simulink model "Grid-Connected Photovoltaic Power System"  (R2024a)
settings: Solver=VariableStepAuto  StartTime=0.0  StopTime=5  RelTol=1e-3
undefined symbols (not defined in the file): D1, Delta
libraries: spsIGBTLib x7, spsThreePhaseVIMeasurementLib x4, spsSeriesRLCBranchLib x3, simulink x3, spsThreePhaseSeriesRLCBranchLib x2, spsThreePhaseTransformerTwoWindingsLib x2, spsVoltageMeasurementLib x2, spsDiodeLib x1, spsGroundLib x1, spsPVArrayLib x1, spsPWMGeneratorDCDCLib x1, spsSawtoothGeneratorLib x1
settings Model: Creator=suresh43  LastModifiedBy=aniru
settings RTWCC: GPUComputeCapability=3.5

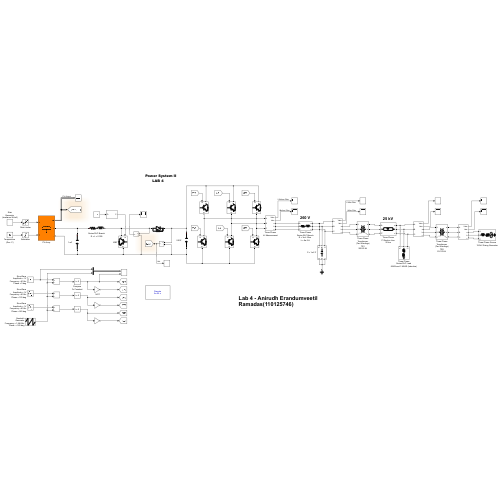
[thumbnail: Simulink's stored preview of the top-level diagram]
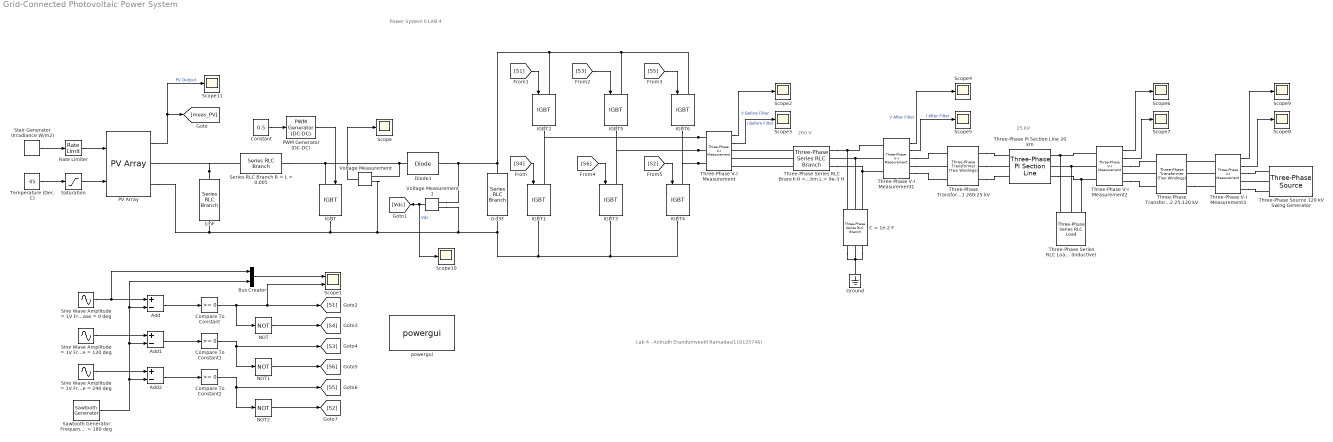
== system Grid-Connected Photovoltaic Power System ==
  note: Power System II
      | LAB 4
  note: 260 V
  note: 25 kV
  note: Lab 4 - Anirudh Erandumveetil Ramadas(110125746)
  0.05F : spsSeriesRLCBranchLib/Series RLC Branch  LConnTagsString=__new0  RConnTagsString=__new0  BranchType=C  Resistance=0  Inductance=0  SetiL0=off  InitialCurrent=0  Capacitance=0.05  Setx0=off  InitialVoltage=0  Measurements=None
  1mF : spsSeriesRLCBranchLib/Series RLC Branch  LConnTagsString=__new0  RConnTagsString=__new0  BranchType=C  Resistance=0  Inductance=0  SetiL0=off  InitialCurrent=0  Capacitance=1e-3  Setx0=off  InitialVoltage=0  Measurements=None
  Add : Sum  Inputs=+-
  Add1 : Sum  Inputs=+-
  Add2 : Sum  Inputs=+-
  Bus Creator : BusCreator  Inputs=2
  C = 1e-2 F : spsThreePhaseSeriesRLCBranchLib/Three-Phase Series RLC Branch  LConnTagsString=A|B|C  RConnTagsString=A|B|C  BranchType=C  Resistance=3e-4  Inductance=9e-5  Capacitance=1e-2  Measurements=None
  Compare To Constant : simulink/Logic and Bit Operations/Compare To Constant  relop=>=  const=0  OutDataTypeStr=boolean
  Compare To Constant1 : simulink/Logic and Bit Operations/Compare To Constant  relop=>=  const=0  OutDataTypeStr=boolean
  Compare To Constant2 : simulink/Logic and Bit Operations/Compare To Constant  relop=>=  const=0  OutDataTypeStr=boolean
  Constant : Constant  Value=0.5
  Diode1 : spsDiodeLib/Diode  Ron=1e-4  Lon=0  Vf=0  IC=0  UseSnubber=0  Rs=500  Cs=250e-9  Measurements=off
  Ground : spsGroundLib/Ground  LConnTagsString=a
  IGBT{,1..6} (7 alike) : spsIGBTLib/IGBT  Ron=0.001  Lon=0  Vf=1  Tf=1e-6  Tt=2e-6  IC=0  Rs=1e5  Cs=inf  Measurements=off
  NOT : Logic  Operator=NOT  IconShape=distinctive  AllPortsSameDT=off  OutDataTypeStr=boolean
  NOT1 : Logic  Operator=NOT  IconShape=distinctive  AllPortsSameDT=off  OutDataTypeStr=boolean
  NOT2 : Logic  Operator=NOT  IconShape=distinctive  AllPortsSameDT=off  OutDataTypeStr=boolean
  PV Array : spsPVArrayLib/PV Array  Npar=48  Nser=7  PlotType=array @ 25 deg.C & specified irradiances  S_vec=[ 1000 ]  Temp_C_vec="[ 45 25  ]"  ModuleName=SunPower SPR-305E-WHT-D  PlotWhenSelected=off  Pm=305.226  Ncell=96  Voc=64.2  Isc=5.96  Vm=54.7  Im=5.58  beta_Voc_pc=-0.2727  alpha_Isc_pc=0.061745  beta_Voc=-0.17507  alpha_Isc=0.00368  IL=5.9657  I0=6.3076e-12  nI=0.94489  Rsh=393.2054  Rs=0.37428  RobustModel=off  RobustCellTemperature=313.3991  BAL=on  Tc=1e-6  Tfilter=5e-5
  PWM Generator (DC-DC) : spsPWMGeneratorDCDCLib/PWM Generator (DC-DC)  Fsw=5e3  Ts=0
  Rate Limiter : RateLimiter  RisingSlewLimit=8000  FallingSlewLimit=-8000  SampleTimeMode=inherited  InitialCondition=1000
  Saturation : Saturate  UpperLimit=55  LowerLimit=5
  Sawtooth Generator Frequency = 1.98 KHz Phase  = 180 deg : spsSawtoothGeneratorLib/Sawtooth Generator  Freq=5000  Phase=180  Ts=0
  Scope{,2..11} (11 alike) : Scope
  Scope1 : Scope  NumInputPorts=2
  Series RLC Branch R = L = 0.005 : spsSeriesRLCBranchLib/Series RLC Branch  LConnTagsString=__new0  RConnTagsString=__new0  BranchType=RL  Resistance=0.005  Inductance=0.005  SetiL0=off  InitialCurrent=0  Capacitance=1e-6  Setx0=off  InitialVoltage=0  Measurements=None
  Sine Wave Amplitude = 1V Frequency = 60 Hz Phase = 0 deg : Sin  Frequency=376.991118  SampleTime=0
  Sine Wave Amplitude = 1V Frequency = 60 Hz Phase = 120 deg : Sin  Frequency=376.991118  Phase=-2.0944  SampleTime=0
  Sine Wave Amplitude = 1V Frequency = 60 Hz Phase = 240 deg : Sin  Frequency=376.991118  Phase=2.0944  SampleTime=0
  Stair Generator (Irradiance W/m2) : spsStairGeneratorLib/Stair Generator  t=[0, 0.4]  e=[0.5, 1]*1000  Ts=5e-5
  Temperature (Dec. C) : Constant  Value=45
  Three-Phase PI Section Line 20 km : spsThreePhasePISectionLineLib/Three-Phase PI Section Line  LConnTagsString=a|b|c  RConnTagsString=A|B|C  Length=20  Frequency=60  Resistances=[ 0.01273 0.3864]  Inductances="[ 0.9337e-3  4.1264e-3]"  Capacitances=[12.74e-9 7.751e-9]
  Three-Phase Series RLC Branch R = 3e-4 Ohm L = 9e-3 H : spsThreePhaseSeriesRLCBranchLib/Three-Phase Series RLC Branch  LConnTagsString=A|B|C  RConnTagsString=A|B|C  BranchType=RL  Resistance=3e-4  Inductance=9e-5  Capacitance=1e-6  Measurements=None
  Three-Phase Series RLC Load 8 MW and 1 MVAR (Inductive) : spsThreePhaseSeriesRLCLoadLib/Three-Phase Series RLC Load  LConnTagsString=A|B|C  Configuration=Y (grounded)  NominalVoltage=25e3  Vabc=[1e3 1e3 1e3]  Vabcp=[1e3 1e3 1e3]  NominalFrequency=60  UnbalancedPower=off  ActivePower=8e6  InductivePower=1e6  CapacitivePower=0  Pabc=[10e3 9e3 11e3]  QLabc=[100 90 110]  QCabc=[100 90 110]  Pabcp=[10e3 9e3 11e3]  QLabcp=[100 90 110]  QCabcp=[100 90 110]  Measurements=None  LoadType=constant Z
  Three-Phase Transformer (Two Windings) TR1 260:25 kV : spsThreePhaseTransformerTwoWindingsLib/Three-Phase Transformer (Two Windings)  Winding1Connection=Delta (D1)  Winding2Connection=Yg  CoreType=Three single-phase transformers  SetSaturation=off  Hysteresis=off  DataFile='hysteresis'  SetInitialFlux=off  Measurements=None  UNITS=pu  NominalPower=[ 100e3 , 60 ]  Winding1=[ 260 , 0.0012 , 0.03 ]  Winding2=[ 25e3 ,0.0012 , 0.03 ]  Rm=500  Lm=500  L0=0.5  Saturation=[ 0,0 ; 0.0024,1.2 ; 1.0,1.52 ]  InitialFluxes=[ 0.8 , -0.8 , 0.7 ]  BreakLoop=off  DiscreteSolver=Trapezoidal iterative  DataType=off  TransfoNumber=1
  Three-Phase Transformer (Two Windings) TR2 25:120 kV : spsThreePhaseTransformerTwoWindingsLib/Three-Phase Transformer (Two Windings)  Winding1Connection=Delta (D1)  Winding2Connection=Yg  CoreType=Three single-phase transformers  SetSaturation=off  Hysteresis=off  DataFile='hysteresis'  SetInitialFlux=off  Measurements=None  UNITS=pu  NominalPower=[ 10e6 , 60 ]  Winding1=[ 25e3 , 0.003 , 0.08 ]  Winding2=[ 120e3 ,0.003 , 0.08 ]  Rm=500  Lm=500  L0=0.5  Saturation=[ 0,0 ; 0.0024,1.2 ; 1.0,1.52 ]  InitialFluxes=[ 0.8 , -0.8 , 0.7 ]  BreakLoop=off  DiscreteSolver=Trapezoidal iterative  DataType=off  TransfoNumber=1
  Three-Phase V-I Measurement{,1..3} (4 alike) : spsThreePhaseVIMeasurementLib/Three-Phase V-I Measurement  VoltageMeasurement=phase-to-ground  SetLabelV=off  LabelV=Vabc  Vpu=off  VpuLL=off  CurrentMeasurement=yes  SetLabelI=off  LabelI=Iabc  Ipu=off  Pbase=100e6  Vbase=500e3  OutputType=Complex  PhasorSimulation=off  PSBequivalent=0
  "Three-Phase Source 120 kV Swing Generator " : spsThreePhaseSourceLib/Three-Phase Source  InternalConnection=Yg  VoltagePhases=off  Voltage=120e3  PhaseAngle=0  Voltage_phases=[25e3 25e3 25e3]/sqrt(3)  PhaseAngles_phases=[0 -120 +120]  Frequency=60  NonIdealSource=on  SpecifyImpedance=on  Resistance=0.8929  Inductance=16.58e-3  ShortCircuitLevel=100e6  BaseVoltage=120e3  XRratio=30  BusType=swing  Pref=10e3  Qref=0  Prefabc=[10e3, 10e3, 10e3]  Qrefabc=[0, 0, 0]  Qmin=-inf  Qmax=inf
  Voltage Measurement : spsVoltageMeasurementLib/Voltage Measurement  PhasorSimulation=off  OutputType=Complex  PSBequivalent=0
  Voltage Measurement1 : spsVoltageMeasurementLib/Voltage Measurement  PhasorSimulation=off  OutputType=Complex  PSBequivalent=0
  powergui : sps_lib/powergui  Priority=1  SimulationMode=Discrete  SampleTime=5e-5  frequency=60  Iterations=50  frequencyindice=0  Pbase=100e6  ErrMax=1e-4  UnitsV=kV  UnitsW=MW  buscounter=0  FunctionMessages=off  echomessages=off  EnableUseOfTLC=off  CurrentSourceSwitches=off  DisableSnubberDevices=off  DisableRonSwitches=off  DisableVfSwitches=off  DisplayEquations=off  AutomaticDiscreteSolvers=off  SolverType=Tustin/Backward Euler (TBE)  Interpol=off  ExternalGateDelay=off  methode=off  Ts=100  x0status=blocks  SPID=on  SwTol=0  HookPort=off  NonlinearTolerance=1e-4  nMaxIteration=100  ContinueOnMaxIteration=off  RestoreLinks=warning  ResistiveCurrentMeasurement=off  Frange=[0:2:500]  Ylog=off  Xlog=on  ShowGrid=off  save=off  variable=ZData  structure=0  ZoomFFT=off  StartTime=0.0  cycles=1  DisplayStyle=1  fundamental=60  FreqAxis=off  MaxFrequency=1000  frequencyindicesteady=1  RmsSteady=1  display=off
  wires:
  Temperature (Dec. C)/1 -> Saturation/1
  Saturation/1 -> PV Array/2
  Stair Generator (Irradiance W/m2)/1 -> Rate Limiter/1
  Rate Limiter/1 -> PV Array/1
  PV Array/1 -> Scope11/1, [meas_PV]  "PV Output"
  Constant/1 -> PWM Generator (DC-DC)/1
  PWM Generator (DC-DC)/1 -> IGBT/1
  Voltage Measurement/1 -> Scope/1
  Voltage Measurement1/1 -> Scope10/1, [Vdc]  "Vdc"
  [S4] -> IGBT1/1
  [S1] -> IGBT2/1
  [S3] -> IGBT5/1
  [S5] -> IGBT6/1
  [S6] -> IGBT3/1
  [S2] -> IGBT4/1
  Sawtooth Generator Frequency = 1.98 KHz Phase  = 180 deg/1 -> Add2/2, Add1/2, Bus Creator/2, Add/2
  Sine Wave Amplitude = 1V Frequency = 60 Hz Phase = 0 deg/1 -> Bus Creator/1, Add/1
  Sine Wave Amplitude = 1V Frequency = 60 Hz Phase = 120 deg/1 -> Add1/1
  Sine Wave Amplitude = 1V Frequency = 60 Hz Phase = 240 deg/1 -> Add2/1
  Add/1 -> Compare To Constant/1
  Add1/1 -> Compare To Constant1/1
  Add2/1 -> Compare To Constant2/1
  Compare To Constant/1 -> Scope1/2, [S1], NOT/1
  Compare To Constant1/1 -> [S3], NOT1/1
  Compare To Constant2/1 -> [S5], NOT2/1
  Bus Creator/1 -> Scope1/1
  NOT/1 -> [S4]
  NOT1/1 -> [S6]
  NOT2/1 -> [S2]
  Three-Phase V-I Measurement/1 -> Scope2/1  "V Before Filter"
  Three-Phase V-I Measurement/2 -> Scope3/1  "I Before Filter"
  Three-Phase V-I Measurement1/1 -> Scope4/1  "V After Filter"
  Three-Phase V-I Measurement1/2 -> Scope5/1  "I After Filter"
  Three-Phase V-I Measurement2/1 -> Scope6/1
  Three-Phase V-I Measurement2/2 -> Scope7/1
  Three-Phase V-I Measurement3/2 -> Scope8/1
  Three-Phase V-I Measurement3/1 -> Scope9/1
  connections:
  1mF/LConn1 -- Series RLC Branch R = L = 0.005/LConn1 -- PV Array/RConn1
  PV Array/RConn2 -- IGBT/RConn1 -- Voltage Measurement1/LConn2 -- IGBT1/RConn1 -- IGBT4/RConn1 -- IGBT3/RConn1 -- 0.05F/RConn1 -- Voltage Measurement/LConn2 -- 1mF/RConn1
  Series RLC Branch R = L = 0.005/RConn1 -- IGBT/LConn1 -- Voltage Measurement/LConn1 -- Diode1/LConn1
  Diode1/RConn1 -- Voltage Measurement1/LConn1 -- IGBT2/LConn1 -- IGBT6/LConn1 -- IGBT5/LConn1 -- 0.05F/LConn1
  Three-Phase V-I Measurement/LConn2 -- IGBT5/RConn1 -- IGBT3/LConn1
  Three-Phase V-I Measurement/LConn1 -- IGBT2/RConn1 -- IGBT1/LConn1
  Three-Phase V-I Measurement/LConn3 -- IGBT6/RConn1 -- IGBT4/LConn1
  Three-Phase Series RLC Branch R = 3e-4 Ohm L = 9e-3 H/LConn3 -- Three-Phase V-I Measurement/RConn3
  Three-Phase Series RLC Branch R = 3e-4 Ohm L = 9e-3 H/LConn2 -- Three-Phase V-I Measurement/RConn2
  Three-Phase Series RLC Branch R = 3e-4 Ohm L = 9e-3 H/LConn1 -- Three-Phase V-I Measurement/RConn1
  Three-Phase V-I Measurement1/LConn2 -- C = 1e-2 F/LConn2 -- Three-Phase Series RLC Branch R = 3e-4 Ohm L = 9e-3 H/RConn2
  Three-Phase Series RLC Branch R = 3e-4 Ohm L = 9e-3 H/RConn1 -- Three-Phase V-I Measurement1/LConn1 -- C = 1e-2 F/LConn1
  Three-Phase Series RLC Branch R = 3e-4 Ohm L = 9e-3 H/RConn3 -- Three-Phase V-I Measurement1/LConn3 -- C = 1e-2 F/LConn3
  Ground/LConn1 -- C = 1e-2 F/RConn3 -- C = 1e-2 F/RConn1 -- C = 1e-2 F/RConn2
  Three-Phase V-I Measurement1/RConn1 -- Three-Phase Transformer (Two Windings) TR1 260:25 kV/LConn1
  Three-Phase V-I Measurement1/RConn2 -- Three-Phase Transformer (Two Windings) TR1 260:25 kV/LConn2
  Three-Phase V-I Measurement1/RConn3 -- Three-Phase Transformer (Two Windings) TR1 260:25 kV/LConn3
  Three-Phase Transformer (Two Windings) TR1 260:25 kV/RConn2 -- Three-Phase PI Section Line 20 km/LConn2
  Three-Phase Transformer (Two Windings) TR1 260:25 kV/RConn1 -- Three-Phase PI Section Line 20 km/LConn1
  Three-Phase Transformer (Two Windings) TR1 260:25 kV/RConn3 -- Three-Phase PI Section Line 20 km/LConn3
  Three-Phase V-I Measurement2/LConn2 -- Three-Phase Series RLC Load 8 MW and 1 MVAR (Inductive)/LConn2 -- Three-Phase PI Section Line 20 km/RConn2
  Three-Phase PI Section Line 20 km/RConn1 -- Three-Phase Series RLC Load 8 MW and 1 MVAR (Inductive)/LConn1 -- Three-Phase V-I Measurement2/LConn1
  Three-Phase PI Section Line 20 km/RConn3 -- Three-Phase Series RLC Load 8 MW and 1 MVAR (Inductive)/LConn3 -- Three-Phase V-I Measurement2/LConn3
  Three-Phase Transformer (Two Windings) TR2 25:120 kV/LConn2 -- Three-Phase V-I Measurement2/RConn2
  Three-Phase V-I Measurement2/RConn1 -- Three-Phase Transformer (Two Windings) TR2 25:120 kV/LConn1
  Three-Phase V-I Measurement2/RConn3 -- Three-Phase Transformer (Two Windings) TR2 25:120 kV/LConn3
  Three-Phase V-I Measurement3/LConn2 -- Three-Phase Transformer (Two Windings) TR2 25:120 kV/RConn2
  Three-Phase V-I Measurement3/LConn1 -- Three-Phase Transformer (Two Windings) TR2 25:120 kV/RConn1
  Three-Phase Transformer (Two Windings) TR2 25:120 kV/RConn3 -- Three-Phase V-I Measurement3/LConn3
  "Three-Phase Source 120 kV Swing Generator "/RConn2 -- Three-Phase V-I Measurement3/RConn2
  Three-Phase V-I Measurement3/RConn1 -- "Three-Phase Source 120 kV Swing Generator "/RConn1
  Three-Phase V-I Measurement3/RConn3 -- "Three-Phase Source 120 kV Swing Generator "/RConn3
